simulink model "dynamics_model_linearize_feedback_281019"  (R2018b)
settings: Solver=VariableStepAuto  StartTime=0.0  StopTime=10.0  RelTol=1e-3
values from neighbouring files (symbols this model uses):
  DIM = data{4}    [gimbal_dynamics.m]
  DIS = data{5}    [gimbal_dynamics.m]
  I1 = data{1}    [gimbal_dynamics.m]    (also in macierze_inercji.m = sym('I1', [4 4]))
  I2 = data{2}    [gimbal_dynamics.m]    (also in macierze_inercji.m = sym('I2', [4 4]))
  I3 = data{3}    [gimbal_dynamics.m]    (also in macierze_inercji.m = sym('I3', [4 4]))
  M = [ud_ucz(3:p-1) ud_ucz(3:p-1).^2 ud_ucz(3:p-1).^3 ud_ucz(2:p-2) ud_ucz(2:p-2).^2 ud_ucz(2:p-2).^3 ud_ucz(1:p-3) ud_ucz(1:p-3).^2 ud_ucz(1:p-3).^3 yd_ucz(3:p-1) yd_ucz(3:p-1).^2 yd_ucz(3:p-1).^3 yd_ucz(2:p-2) yd_ucz(2:p-2).^2 yd_ucz(2:p-2).^3 yd_ucz(1:p-3) yd_ucz(1:p-3).^2 yd_ucz(1:p-3).^3]    [Identification_20191023.m]    (also in MI_beta.m = fillmissing(M,'spline'); gimbal_dynamics.m = data{6}; macierze_inercji.m = sym('M', [1 3]))
libraries: simulink x2
settings Model: Creator=Paweł Tymiński  LastModifiedBy=Paweł Tymiński

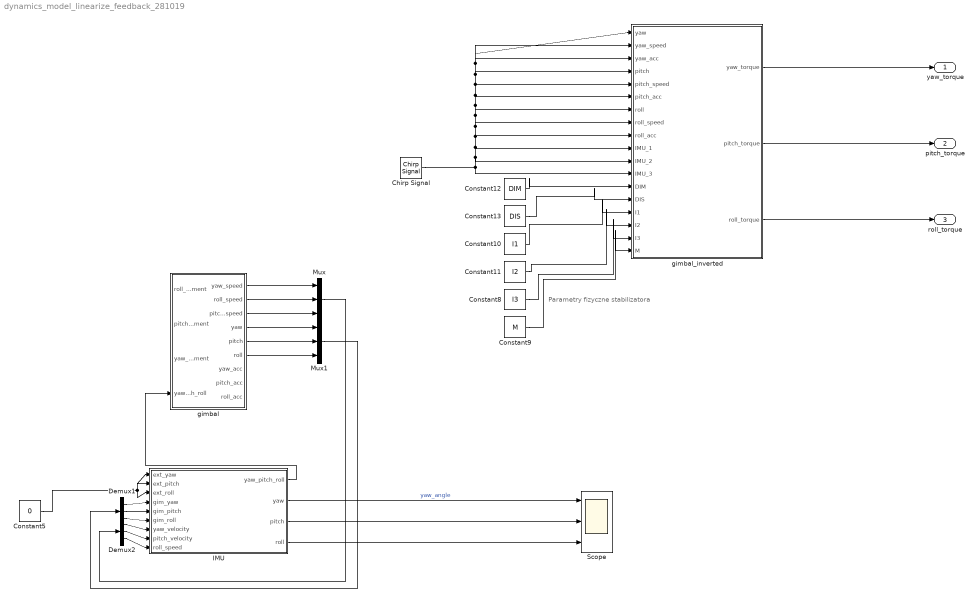
== system dynamics_model_linearize_feedback_281019 ==
  note: Parametry fizyczne stabilizatora
  Chirp Signal : simulink/Sources/Chirp Signal  f1=1  T=100  f2=20
  Constant10 : Constant  Value=I1
  Constant11 : Constant  Value=I2
  Constant12 : Constant  Value=DIM
  Constant13 : Constant  Value=DIS
  Constant5 : Constant  Value=0
  Constant8 : Constant  Value=I3
  Constant9 : Constant  Value=M
  Demux1 : Demux  Outputs=3
  Demux2 : Demux  Outputs=3
  IMU : Subsystem
  Mux : Mux  Inputs=3
  Mux1 : Mux  Inputs=3
  Scope : Scope  NumInputPorts=3
  gimbal : Subsystem
  gimbal_inverted : MATLAB Function  TreatAsAtomicUnit=on
  yaw_torque : Outport
  pitch_torque : Outport  Port=2
  roll_torque : Outport  Port=3
  wires:
  Demux1/2 -> IMU/5(gim_pitch)
  gimbal/5(pitch) -> Mux1/2
  Demux2/1 -> IMU/7(yaw_velocity)
  IMU/3(pitch) -> Scope/2
  Demux1/1 -> IMU/4(gim_yaw)
  IMU/4(roll) -> Scope/3
  Demux2/3 -> IMU/9(roll_speed)
  Demux2/2 -> IMU/8(pitch_velocity)
  gimbal/4(yaw) -> Mux1/1
  Demux1/3 -> IMU/6("gim_roll ")
  gimbal/3(pitch_speed) -> Mux/3
  gimbal/2(roll_speed) -> Mux/2
  Mux1/1 -> Demux1/1
  IMU/1(yaw_pitch_roll) -> gimbal/4(yaw_pitch_roll)
  Mux/1 -> Demux2/1
  gimbal/6(roll) -> Mux1/3
  IMU/2(yaw) -> Scope/1  "yaw_angle"
  Constant5/1 -> IMU/3(ext_roll), IMU/1(ext_yaw), IMU/2(ext_pitch)
  gimbal/1(yaw_speed) -> Mux/1
  gimbal_inverted/3(roll_torque) -> roll_torque/1
  gimbal_inverted/2(pitch_torque) -> pitch_torque/1
  Constant13/1 -> gimbal_inverted/14(DIS)
  Constant10/1 -> gimbal_inverted/15(I1)
  gimbal_inverted/1(yaw_torque) -> yaw_torque/1
  Chirp Signal/1 -> gimbal_inverted/4(pitch), gimbal_inverted/1(yaw), gimbal_inverted/2(yaw_speed), gimbal_inverted/3(yaw_acc), gimbal_inverted/5(pitch_speed), gimbal_inverted/6(pitch_acc), gimbal_inverted/7(roll), gimbal_inverted/8(roll_speed), gimbal_inverted/9(roll_acc), gimbal_inverted/10(IMU_1), gimbal_inverted/11(IMU_2), gimbal_inverted/12(IMU_3)
  Constant8/1 -> gimbal_inverted/17(I3)
  Constant9/1 -> gimbal_inverted/18(M)
  Constant12/1 -> gimbal_inverted/13(DIM)
  Constant11/1 -> gimbal_inverted/16(I2)

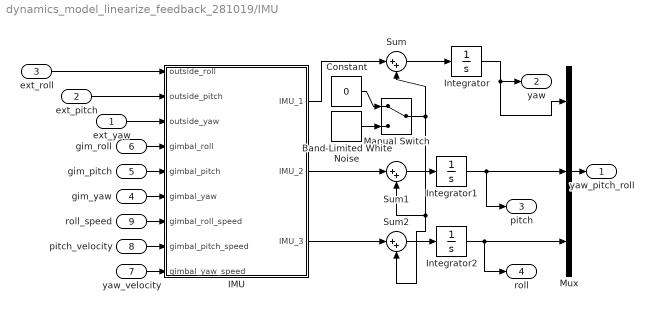
== system dynamics_model_linearize_feedback_281019/IMU ==
  ext_yaw : Inport
  ext_pitch : Inport  Port=2
  ext_roll : Inport  Port=3
  gim_yaw : Inport  Port=4
  gim_pitch : Inport  Port=5
  "gim_roll " : Inport  Port=6
  yaw_velocity : Inport  Port=7
  pitch_velocity : Inport  Port=8
  roll_speed : Inport  Port=9
  Band-Limited White Noise : simulink/Sources/Band-Limited White Noise  Cov=[0.1]  Ts=0.1  seed=[23341]
  Constant : Constant  Value=0
  IMU : MATLAB Function  TreatAsAtomicUnit=on
  Integrator : Integrator
  Integrator1 : Integrator
  Integrator2 : Integrator
  Manual Switch : ManualSwitch
  Mux : Mux  Inputs=3
  Sum : Sum  Inputs=|++
  Sum1 : Sum  Inputs=|++
  Sum2 : Sum  Inputs=|++
  yaw_pitch_roll : Outport
  yaw : Outport  Port=2
  pitch : Outport  Port=3
  roll : Outport  Port=4
  wires:
  roll_speed/1 -> IMU/7(gimbal_roll_speed)
  gim_pitch/1 -> IMU/5(gimbal_pitch)
  Mux/1 -> yaw_pitch_roll/1
  yaw_velocity/1 -> IMU/9(gimbal_yaw_speed)
  IMU/1(IMU_1) -> Sum/1
  pitch_velocity/1 -> IMU/8(gimbal_pitch_speed)
  ext_pitch/1 -> IMU/2(outside_pitch)
  ext_roll/1 -> IMU/1(outside_roll)
  ext_yaw/1 -> IMU/3(outside_yaw)
  "gim_roll "/1 -> IMU/4(gimbal_roll)
  gim_yaw/1 -> IMU/6(gimbal_yaw)
  IMU/3(IMU_3) -> Sum2/1
  IMU/2(IMU_2) -> Sum1/1
  Integrator2/1 -> roll/1, Mux/3
  Manual Switch/1 -> Sum2/2, Sum1/2, Sum/2
  Sum2/1 -> Integrator2/1
  Sum1/1 -> Integrator1/1
  Sum/1 -> Integrator/1
  Integrator1/1 -> pitch/1, Mux/2
  Integrator/1 -> yaw/1, Mux/1
  Band-Limited White Noise/1 -> Manual Switch/2
  Constant/1 -> Manual Switch/1

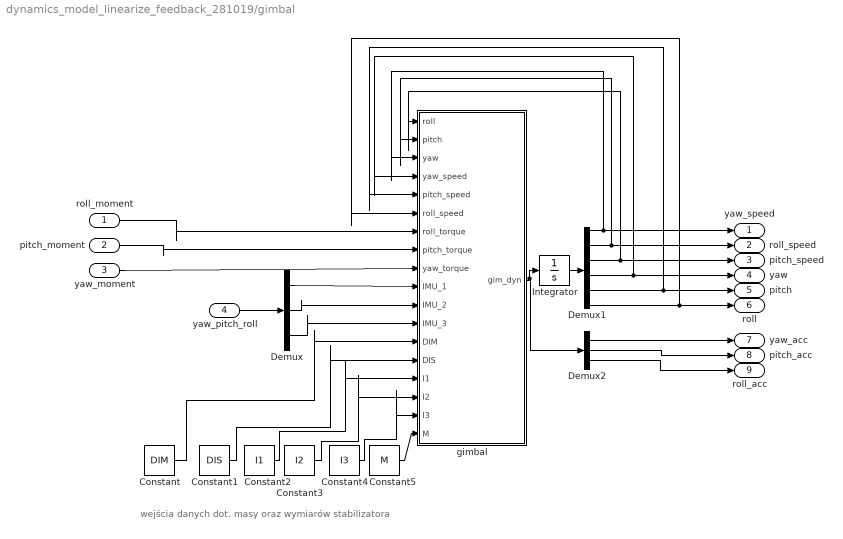
== system dynamics_model_linearize_feedback_281019/gimbal ==
  note: wejścia danych dot. masy oraz wymiarów stabilizatora
  roll_moment : Inport
  pitch_moment : Inport  Port=2
  yaw_moment : Inport  Port=3
  yaw_pitch_roll : Inport  Port=4
  Constant : Constant  Value=DIM
  Constant1 : Constant  Value=DIS
  Constant2 : Constant  Value=I1
  Constant3 : Constant  Value=I2
  Constant4 : Constant  Value=I3
  Constant5 : Constant  Value=M
  Demux : Demux  Outputs=3
  Demux1 : Demux  Outputs=6
  Demux2 : Demux  Outputs=3
  Integrator : Integrator
  gimbal : MATLAB Function  TreatAsAtomicUnit=on
  yaw_speed : Outport
  roll_speed : Outport  Port=2
  pitch_speed : Outport  Port=3
  yaw : Outport  Port=4
  pitch : Outport  Port=5
  roll : Outport  Port=6
  yaw_acc : Outport  Port=7
  pitch_acc : Outport  Port=8
  roll_acc : Outport  Port=9
  wires:
  Demux/1 -> gimbal/10(IMU_1)
  Demux/3 -> gimbal/12(IMU_3)
  Demux/2 -> gimbal/11(IMU_2)
  gimbal/1(gim_dyn) -> Demux2/1, Integrator/1
  Demux1/2 -> roll_speed/1, gimbal/2(pitch)
  Demux1/1 -> yaw_speed/1, gimbal/3(yaw)
  yaw_pitch_roll/1 -> Demux/1
  Demux1/5 -> gimbal/5(pitch_speed), pitch/1
  Demux1/6 -> gimbal/6(roll_speed), roll/1
  roll_moment/1 -> gimbal/7(roll_torque)
  Demux1/4 -> gimbal/4(yaw_speed), yaw/1
  yaw_moment/1 -> gimbal/9(yaw_torque)
  pitch_moment/1 -> gimbal/8(pitch_torque)
  Demux1/3 -> pitch_speed/1, gimbal/1(roll)
  Integrator/1 -> Demux1/1
  Constant5/1 -> gimbal/18(M)
  Constant4/1 -> gimbal/17(I3)
  Constant3/1 -> gimbal/16(I2)
  Constant2/1 -> gimbal/15(I1)
  Constant1/1 -> gimbal/14(DIS)
  Constant/1 -> gimbal/13(DIM)
  Demux2/1 -> yaw_acc/1
  Demux2/2 -> pitch_acc/1
  Demux2/3 -> roll_acc/1

== matlab function dynamics_model_linearize_feedback_281019/IMU/IMU ==
  data: outside_roll input; IMU_1 output; outside_pitch input; outside_yaw input; gimbal_roll input; gimbal_pitch input; gimbal_yaw input; gimbal_roll_speed input; gimbal_pitch_speed input; gimbal_yaw_speed input; IMU_2 output; IMU_3 output

function [IMU_1, IMU_2, IMU_3] = IMU(outside_roll,outside_pitch,outside_yaw,gimbal_roll , gimbal_pitch , gimbal_yaw , gimbal_roll_speed ,gimbal_pitch_speed , gimbal_yaw_speed )
% kąty gimbala
theta_1 = gimbal_yaw ;
theta_2 = gimbal_pitch ;
theta_3 = gimbal_roll ;

J_0 =[1 0 0;
    0 cos(theta_1) -sin(theta_1);
   -sin(theta_2) cos(theta_2)*sin(theta_1) cos(theta_1)*cos(theta_2)];
Phi_0 = [outside_yaw; outside_pitch; outside_roll];

Omega_phi = J_0*Phi_0;

Omega = [gimbal_yaw_speed; gimbal_pitch_speed; gimbal_roll_speed];

J = [cos(theta_2)*cos(theta_3) sin(theta_3) 0;
    cos(theta_2)*sin(theta_3) cos(theta_3) 0;
    -sin(theta_2) 0 1];
A=J*(Omega_phi + Omega);

IMU_1 = A(1); %yaw
IMU_2 = A(2); %pitch
IMU_3 = A(3); %roll

end

== matlab function dynamics_model_linearize_feedback_281019/gimbal/gimbal ==
  data: roll input; gim_dyn output; pitch input; yaw input; yaw_speed input; pitch_speed input; roll_speed input; roll_torque input; pitch_torque input; yaw_torque input; IMU_1 input; IMU_2 input; IMU_3 input; DIM input; DIS input; I1 input; I2 input; I3 input; M input
%Opis dynamiki stabilizatora w oparciu o wzory wyprowadzone z pracy
%"Stephan von Nispen - Design and control of a three-axis gimbal"



function gim_dyn = gimbal_dynamics(roll,pitch,yaw,yaw_speed,pitch_speed,roll_speed,roll_torque,pitch_torque,yaw_torque,IMU_1,IMU_2,IMU_3,DIM,DIS,I1,I2,I3,M)

%stała grawitacji
g = 9.81;


%-------------ZMIENNE--------------
% odczyty z IMU
alpha_1 = IMU_1;
alpha_2 = IMU_2;
alpha_3 = IMU_3;
IMU = [alpha_1; alpha_2; alpha_3];

% momenty generowane przez silnik - zmienne sterujace
 T1 = yaw_torque ;
 T2 = pitch_torque ;
 T3 = roll_torque ;
%predkosci katowe osiagane przez gimbal
 om_1 = yaw_speed ;
 om_2 = pitch_speed ;
 om_3 = roll_speed ;
Omega = [om_1; om_2; om_3];
%kąty osiagane aktualnie przez gimbal
 theta_1 = yaw ;
 theta_2 = pitch ;
 theta_3 = roll ;
    THETA = [theta_1; theta_2; theta_3];

%---------------FUNKCJE---------------------

H = calculate_H_matrix(THETA,Omega,I1,I2,I3,DIM);
D = calculate_D_matrix(THETA,I1,I2,I3,DIM);
Q = calculate_Q_matrix(T1,T2,T3,Omega);
G = calculate_G_matrix(IMU,THETA,DIM,g,M,DIS);

gim_dyn = [inv(D)\(Q-H-G); Omega];
end

== matlab function dynamics_model_linearize_feedback_281019/gimbal_inverted ==
  data: yaw input; yaw_speed input; yaw_acc input; pitch input; pitch_speed input; pitch_acc input; roll input; yaw_torque output; roll_speed input; roll_acc input; IMU_1 input; IMU_2 input; IMU_3 input; DIM input; DIS input; I1 input; I2 input; I3 input; M input; pitch_torque output; roll_torque output
function [yaw_torque, pitch_torque, roll_torque]  = gimbal_dynamics(yaw,yaw_speed,yaw_acc,pitch,pitch_speed,pitch_acc,roll,roll_speed, roll_acc,IMU_1,IMU_2,IMU_3,DIM,DIS,I1,I2,I3,M)

%stała grawitacji
g = 9.81;


%-------------ZMIENNE--------------
% odczyty z IMU
alpha_1 = IMU_1;
alpha_2 = IMU_2;
alpha_3 = IMU_3;
IMU = [alpha_1; alpha_2; alpha_3];
%predkosci katowe osiagane przez gimbal
 om_1 = yaw_speed ;
 om_2 = pitch_speed ;
 om_3 = roll_speed ;
Omega = [om_1; om_2; om_3];
%kąty osiagane aktualnie przez gimbal
 theta_1 = yaw ;
 theta_2 = pitch ;
 theta_3 = roll ;
 THETA = [theta_1; theta_2; theta_3];
% przyśpieszenia kątowe w osiach gimbala
 ACC = [yaw_acc;pitch_acc;roll_acc];

%---------------FUNKCJE---------------------

H = calculate_H_matrix(THETA,Omega,I1,I2,I3,DIM);
D = calculate_D_matrix(THETA,I1,I2,I3,DIM);
G = calculate_G_matrix(IMU,THETA,DIM,g,M,DIS);
Q = D*ACC+H+G;
yaw_torque = Q(1);
pitch_torque = Q(2);
roll_torque = Q(3);

end
